simulink model "Wishbone_loads"  (R2024b)
settings: Solver=VariableStepAuto  StartTime=0.0  StopTime=10.0  RelTol=1e-3
libraries: simulink x6
(part 1 of 2)
settings Model: Creator=andre  LastModifiedBy=andre

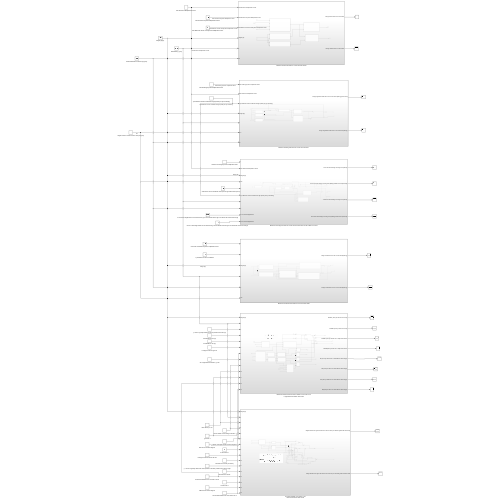
[thumbnail: Simulink's stored preview of the top-level diagram]
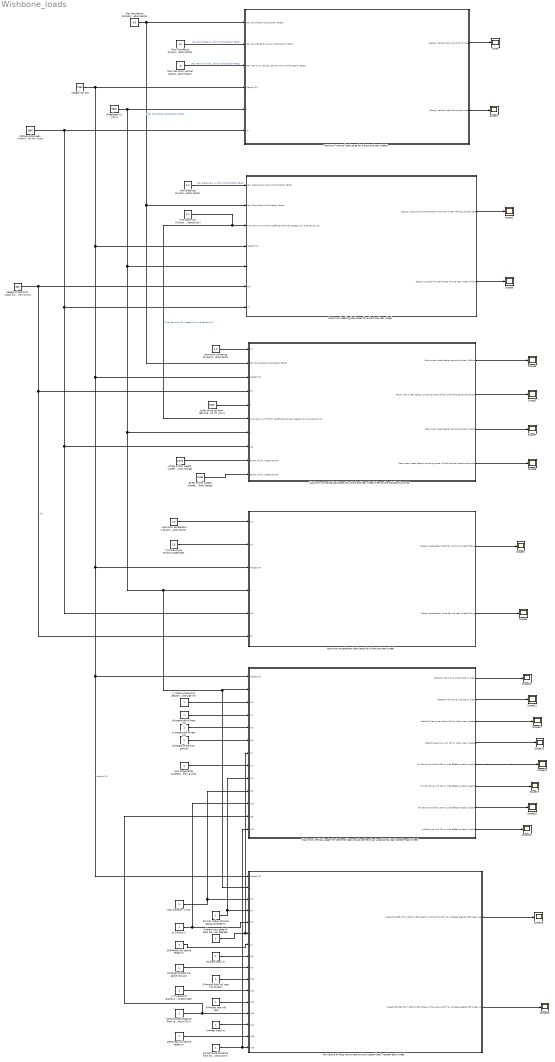
== system Wishbone_loads ==
  37.5% of this weight tranfer can be assumed to go to rear wheels nned to figure out where this comes from though : Constant  Value=0.375
  62.5% of this weight tranfer can be assumed to go to front wheels nned to figure out where this comes from though : Constant  Value=0.625
  Alpha= max angle of bank from floor degrees : Constant
  Ax= longitudinal acceleration  g units : Constant
  Distance Between Front Axle (lm) [mm] : Constant  Value=1950
  For Centre of Mass not at centre of car Lateral load Transfer-each wheel : Subsystem
  H=height of total CG above roll axis : Constant
  Height of centre of mass from the road (Hm) [mm] : Constant  Value=325
  KF=total front roll rate ( lb.-ft/rad?) : Constant
  KR=total rear roll rate : Constant
  Max Breaking Dynamic Multiplication Factor : Constant  Value=1.3
  Max Downforce Dynamic Multiplication Factor : Constant  Value=1.3
  Max Downforce Multiplication Factor : Constant  Value=3.3
  Max Maximum Verical Load Dynamic Multiplication Factor : Constant  Value=3
  Max Velocity- V m/s : Constant
  "Maximum Vertical Loads-For Centre of Mass not at centre of car Longitudinal load transfer-each wheel " : Subsystem
  Maximum acceleraton load cases for a front and rear wheel : Subsystem
  Maximum breaking load cases for a front and rear wheel : Subsystem
  Maximum cornering load cases for a front and rear wheel when on the outside of a corner : Subsystem
  Maximum vertical load cases for a front and rear wheels : Subsystem
  R=max radius of circle being cornered m : Constant
  Scope{,1..19} (20 alike) : Scope
  Tyre Maximum Friction Coefficient : Constant  Value=1.5
  Tyre Maximum Friction Coefficient at high speeds (low tyre sensitivity) : Constant  Value=1.2
  Weight (W) [N] : Constant  Value=7350
  Wheelbase (L) [mm] : Constant  Value=3215
  ZRF=front roll centre height m : Constant
  ZRR=rear roll centre height m : Constant
  a=horizontal distance from front axle to CG m : Constant
  b=horizontal distance from rear axle to CG m : Constant
  g- 9.81ms-2 : Constant
  "h=height of CG from ground " : Constant
  maximum acceleration Dynamic multiplication factor : Constant  Value=1.3
  maximum cornering Dynamic multiplication factor : Constant  Value=1.3
  tf treadwidth of front (m) : Constant
  tf=front track m : Constant
  tr treadwidth of rear (m) : Constant
  tr=rear track m : Constant
  width of the car from left wheel centre point to right wheel centre point (T) [mm] : Constant  Value=1500
  y’’ centre of gravitys offset from centre position to the side (m) : Constant
  "y’’= centre of gravitys offset from centre position to the side, positive when going to right" : Constant
  wires:
  Max Downforce Dynamic Multiplication Factor/1 -> Maximum vertical load cases for a front and rear wheels/2(Max Downforce Dynamic Multiplication Factor)  "Max Downforce Dynamic Multiplication Factor"
  Max Maximum Verical Load Dynamic Multiplication Factor/1 -> Maximum vertical load cases for a front and rear wheels/3(Max Maximum Verical Load Dynamic Multiplication Factor)  "Max Maximum Verical Load Dynamic Multiplication Factor"
  Weight (W) [N]/1 -> Maximum vertical load cases for a front and rear wheels/4(Weight (W)), Maximum breaking load cases for a front and rear wheel/4(Weight (W)), For Centre of Mass not at centre of car Lateral load Transfer-each wheel/1(Weight (W)), "Maximum Vertical Loads-For Centre of Mass not at centre of car Longitudinal load transfer-each wheel "/1(Weight (W)), Maximum acceleraton load cases for a front and rear wheel/3(Weight (W)), Maximum cornering load cases for a front and rear wheel when on the outside of a corner/3(Weight (W))  "Weight (W)"
  Wheelbase (L) [mm]/1 -> For Centre of Mass not at centre of car Lateral load Transfer-each wheel/2(L), "Maximum Vertical Loads-For Centre of Mass not at centre of car Longitudinal load transfer-each wheel "/2(L), Maximum acceleraton load cases for a front and rear wheel/4(L), Maximum cornering load cases for a front and rear wheel when on the outside of a corner/7(L), Maximum breaking load cases for a front and rear wheel/5(L), Maximum vertical load cases for a front and rear wheels/5(L)  "L"
  Distance Between Front Axle (lm) [mm]/1 -> Maximum acceleraton load cases for a front and rear wheel/5(In5), Maximum cornering load cases for a front and rear wheel when on the outside of a corner/8(In8), Maximum breaking load cases for a front and rear wheel/7(lm), Maximum vertical load cases for a front and rear wheels/6(lm)
  Maximum vertical load cases for a front and rear wheels/1(Design Vertical load of one front wheel) -> Scope/1
  Maximum vertical load cases for a front and rear wheels/2(Design Vertical load of one rear wheel) -> Scope4/1
  Max Downforce Multiplication Factor/1 -> Maximum cornering load cases for a front and rear wheel when on the outside of a corner/2(Max Downforce Multiplication Factor), Maximum breaking load cases for a front and rear wheel/2(Max Downforce Multiplication Factor), Maximum vertical load cases for a front and rear wheels/1(Max Downforce Multiplication Factor)  "Max Downforce Multiplication Factor"
  Max Breaking Dynamic Multiplication Factor/1 -> Maximum breaking load cases for a front and rear wheel/1(Max breaking dynamic multiplication factor)  "Max breaking dynamic multiplication factor"
  Tyre Maximum Friction Coefficient at high speeds (low tyre sensitivity)/1 -> Maximum cornering load cases for a front and rear wheel when on the outside of a corner/6(Tyre Maximum Friction Coefficient at high speeds (low tyre sensitivity)), Maximum breaking load cases for a front and rear wheel/3(Tyre Maximum Friction Coefficient at high speeds (low tyre sensitivity))  "Tyre Maximum Friction Coefficient at high speeds (low tyre sensitivity)"
  Height of centre of mass from the road (Hm) [mm]/1 -> Maximum acceleraton load cases for a front and rear wheel/6(Hm), Maximum cornering load cases for a front and rear wheel when on the outside of a corner/4(Hm), Maximum breaking load cases for a front and rear wheel/6(Hm)  "Hm"
  Maximum breaking load cases for a front and rear wheel/1(Design longitudinal brake force for one front wheel (Wflong) [critical case]) -> Scope1/1
  Maximum breaking load cases for a front and rear wheel/2(Design longitudinal brake force for one rear wheel (Wrlong)) -> Scope5/1
  maximum cornering Dynamic multiplication factor/1 -> Maximum cornering load cases for a front and rear wheel when on the outside of a corner/1(In1)
  width of the car from left wheel centre point to right wheel centre point (T) [mm]/1 -> Maximum cornering load cases for a front and rear wheel when on the outside of a corner/5(T)
  Maximum cornering load cases for a front and rear wheel when on the outside of a corner/1(Front outer wheel design cornering force (Wfolat)) -> Scope6/1
  Maximum cornering load cases for a front and rear wheel when on the outside of a corner/4(Rear outer wheel design cornering force (Wrilat) [smaller force expericned]) -> Scope8/1
  Maximum cornering load cases for a front and rear wheel when on the outside of a corner/3(Rear outer wheel design cornering force (Wrolat)) -> Scope7/1
  Maximum cornering load cases for a front and rear wheel when on the outside of a corner/2(Front inner wheel design cornering force (Wfilat) [smaller forces experienced]) -> Scope2/1
  maximum acceleration Dynamic multiplication factor/1 -> Maximum acceleraton load cases for a front and rear wheel/1(In1)
  Tyre Maximum Friction Coefficient/1 -> Maximum acceleraton load cases for a front and rear wheel/2(In2)
  Maximum acceleraton load cases for a front and rear wheel/1(Design acceleration force for one front wheel(Wflong)) -> Scope3/1
  Maximum acceleraton load cases for a front and rear wheel/2(Design acceleration force for one rear wheel(Wrlong)) -> Scope9/1
  37.5% of this weight tranfer can be assumed to go to rear wheels nned to figure out where this comes from though/1 -> Maximum cornering load cases for a front and rear wheel when on the outside of a corner/9("37.5% of this weight tranfer ")
  62.5% of this weight tranfer can be assumed to go to front wheels nned to figure out where this comes from though/1 -> Maximum cornering load cases for a front and rear wheel when on the outside of a corner/10(62.5% of this weight tranfer)
  y’’ centre of gravitys offset from centre position to the side (m)/1 -> "Maximum Vertical Loads-For Centre of Mass not at centre of car Longitudinal load transfer-each wheel "/3(In3)
  tf treadwidth of front (m)/1 -> "Maximum Vertical Loads-For Centre of Mass not at centre of car Longitudinal load transfer-each wheel "/4(In4)
  tr treadwidth of rear (m)/1 -> "Maximum Vertical Loads-For Centre of Mass not at centre of car Longitudinal load transfer-each wheel "/5(In5)
  "h=height of CG from ground "/1 -> "Maximum Vertical Loads-For Centre of Mass not at centre of car Longitudinal load transfer-each wheel "/6(In6)
  Ax= longitudinal acceleration  g units/1 -> "Maximum Vertical Loads-For Centre of Mass not at centre of car Longitudinal load transfer-each wheel "/8(In7)
  "Maximum Vertical Loads-For Centre of Mass not at centre of car Longitudinal load transfer-each wheel "/1(DeltaW1 (front tyre without CG on side)) -> Scope10/1
  "Maximum Vertical Loads-For Centre of Mass not at centre of car Longitudinal load transfer-each wheel "/2(DeltaW2 (front tyre with CG on side)) -> Scope11/1
  "Maximum Vertical Loads-For Centre of Mass not at centre of car Longitudinal load transfer-each wheel "/3(DeltaW3 (rear tyre without CG on side) load increase) -> Scope12/1
  "Maximum Vertical Loads-For Centre of Mass not at centre of car Longitudinal load transfer-each wheel "/4(DeltaW4(rear tyre with CG on side) load increase) -> Scope13/1
  Max Velocity- V m/s/1 -> "Maximum Vertical Loads-For Centre of Mass not at centre of car Longitudinal load transfer-each wheel "/10(In9), For Centre of Mass not at centre of car Lateral load Transfer-each wheel/3(In3)
  R=max radius of circle being cornered m/1 -> "Maximum Vertical Loads-For Centre of Mass not at centre of car Longitudinal load transfer-each wheel "/9(In2), For Centre of Mass not at centre of car Lateral load Transfer-each wheel/4(In4)
  Alpha= max angle of bank from floor degrees/1 -> "Maximum Vertical Loads-For Centre of Mass not at centre of car Longitudinal load transfer-each wheel "/7(In1), For Centre of Mass not at centre of car Lateral load Transfer-each wheel/6(u)
  ZRF=front roll centre height m/1 -> For Centre of Mass not at centre of car Lateral load Transfer-each wheel/7(In7)
  tf=front track m/1 -> For Centre of Mass not at centre of car Lateral load Transfer-each wheel/8(In8)
  H=height of total CG above roll axis/1 -> For Centre of Mass not at centre of car Lateral load Transfer-each wheel/9(In9)
  KF=total front roll rate ( lb.-ft/rad?)/1 -> For Centre of Mass not at centre of car Lateral load Transfer-each wheel/10(In10)
  "y’’= centre of gravitys offset from centre position to the side, positive when going to right"/1 -> For Centre of Mass not at centre of car Lateral load Transfer-each wheel/11(In11)
  KR=total rear roll rate/1 -> For Centre of Mass not at centre of car Lateral load Transfer-each wheel/12(In12)
  b=horizontal distance from rear axle to CG m/1 -> "Maximum Vertical Loads-For Centre of Mass not at centre of car Longitudinal load transfer-each wheel "/12(In8), For Centre of Mass not at centre of car Lateral load Transfer-each wheel/13(In13)
  tr=rear track m/1 -> For Centre of Mass not at centre of car Lateral load Transfer-each wheel/14(In14)
  ZRR=rear roll centre height m/1 -> For Centre of Mass not at centre of car Lateral load Transfer-each wheel/15(In15)
  For Centre of Mass not at centre of car Lateral load Transfer-each wheel/1(Weight transfer from right to left wheel on the front axle(+ve indicates greater left wheel load)) -> Scope18/1
  For Centre of Mass not at centre of car Lateral load Transfer-each wheel/2(Weight transfer from right to left wheel on the rear axle(+ve indicates greater left wheel load) -> Scope19/1
  g- 9.81ms-2/1 -> "Maximum Vertical Loads-For Centre of Mass not at centre of car Longitudinal load transfer-each wheel "/11(In11), For Centre of Mass not at centre of car Lateral load Transfer-each wheel/5(In5)
  a=horizontal distance from front axle to CG m/1 -> "Maximum Vertical Loads-For Centre of Mass not at centre of car Longitudinal load transfer-each wheel "/13(In12), For Centre of Mass not at centre of car Lateral load Transfer-each wheel/16(In16)
  "Maximum Vertical Loads-For Centre of Mass not at centre of car Longitudinal load transfer-each wheel "/5(W1 (front tyre without CG on side Effective static weight)) -> Scope14/1
  "Maximum Vertical Loads-For Centre of Mass not at centre of car Longitudinal load transfer-each wheel "/6(W2 (front tyre with CG on side effective static weight)) -> Scope17/1
  "Maximum Vertical Loads-For Centre of Mass not at centre of car Longitudinal load transfer-each wheel "/7(W3 (rear tyre without CG on side effective static weight)) -> Scope16/1
  "Maximum Vertical Loads-For Centre of Mass not at centre of car Longitudinal load transfer-each wheel "/8(W4(rear tyre with CG on side effective static weight)) -> Scope15/1

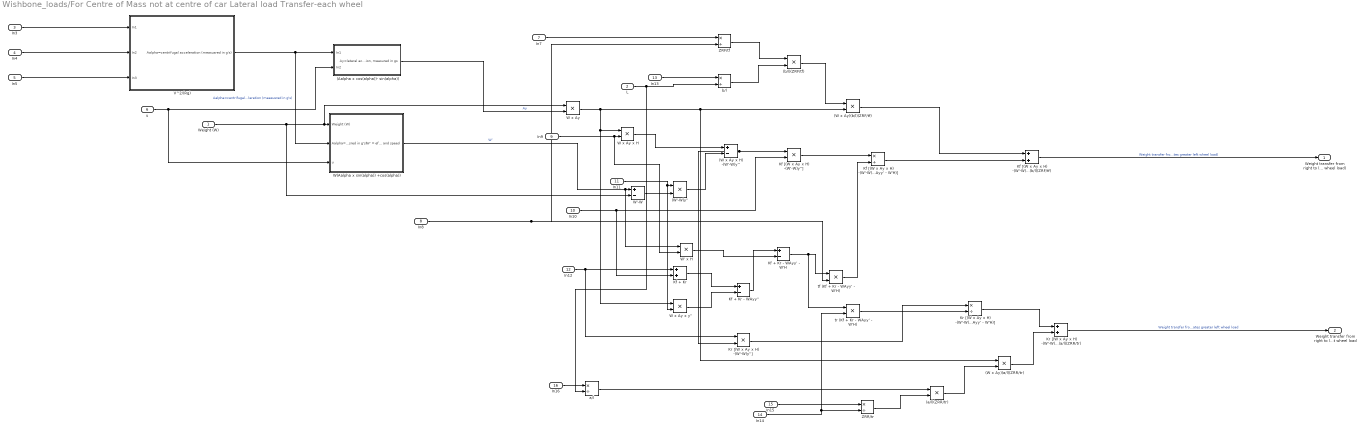
== system Wishbone_loads/For Centre of Mass not at centre of car Lateral load Transfer-each wheel ==
  Weight (W) : Inport
  L : Inport  Port=2
  In3 : Inport  Port=3
  In4 : Inport  Port=4
  In5 : Inport  Port=5
  u : Inport  Port=6
  In7 : Inport  Port=7
  In8 : Inport  Port=8
  In9 : Inport  Port=9
  In10 : Inport  Port=10
  In11 : Inport  Port=11
  In12 : Inport  Port=12
  In13 : Inport  Port=13
  In14 : Inport  Port=14
  In15 : Inport  Port=15
  In16 : Inport  Port=16
  (Aalpha x cos(alpha))- sin(alpha)) : Subsystem
  (W x Ay x H) -(W'-W)y'' : Sum  Inputs=+-
  (W x Ay)(a/l)(ZRR/tr) : Product
  (W x Ay)(b/l)(ZRF/tf) : Product
  (W'-W)y'' : Product
  (a/l)(ZRR/tr) : Product
  (b/l)(ZRF/tf) : Product
  Kf + Kr : Sum
  Kf + Kr - WAyy' - W'H : Sum  Inputs=+-
  Kf + Kr - WAyy'' : Sum  Inputs=+-
  Kf [(W x Ay x H) -(W'-W)y''] : Product
  Kf [(W x Ay x H) -(W'-W)y''] / [tf (Kf + Kr - WAyy' - W'H)] : Product  Inputs=*/
  Kf [(W x Ay x H) -(W'-W)y''] / [tf (Kf + Kr - WAyy' - W'H)] + (W x Ay)(b/l)(ZRF/tf) : Sum
  Kr [(W x Ay x H) -(W'-W)y''] : Product
  Kr [(W x Ay x H) -(W'-W)y''] / [tr (Kf + Kr - WAyy' - W'H)] : Product  Inputs=*/
  Kr [(W x Ay x H) -(W'-W)y''] / [tr (Kf + Kr - WAyy' - W'H)]/ (W x Ay)(a/l)(ZRR/tr) : Sum
  V^2/(Rg) : Subsystem
  W x Ay : Product
  W x Ay x H : Product
  W x Ay x y'' : Product
  W' x H : Product
  W'-W : Sum  Inputs=+-
  W(Aalpha x sin(alpha)) +cos(alpha)) : Subsystem
  ZRF/tf : Product  Inputs=*/
  ZRR/tr : Product  Inputs=*/
  a/l : Product  Inputs=*/
  b/l : Product  Inputs=*/
  tf (Kf + Kr - WAyy' - W'H) : Product
  tr (Kf + Kr - WAyy' - W'H) : Product
  Weight transfer from right to left wheel on the front axle(+ve indicates greater left wheel load) : Outport
  Weight transfer from right to left wheel on the rear axle(+ve indicates greater left wheel load : Outport  Port=2
  wires:
  Kr [(W x Ay x H) -(W'-W)y'']/1 -> Kr [(W x Ay x H) -(W'-W)y''] / [tr (Kf + Kr - WAyy' - W'H)]/1
  ZRR/tr/1 -> (a/l)(ZRR/tr)/2
  Weight (W)/1 -> W'-W/2, W x Ay/1, W(Aalpha x sin(alpha)) +cos(alpha))/1(Weight (W))
  In5/1 -> V^2/(Rg)/3(In3)
  Kf [(W x Ay x H) -(W'-W)y'']/1 -> Kf [(W x Ay x H) -(W'-W)y''] / [tf (Kf + Kr - WAyy' - W'H)]/1
  V^2/(Rg)/1(Aalpha=centrifugal acceleration (measusred in g's)) -> W(Aalpha x sin(alpha)) +cos(alpha))/2(Aalpha=centrifugal acceleration (measusred in g's)), (Aalpha x cos(alpha))- sin(alpha))/1(In1)  "Aalpha=centrifugal acceleration (measusred in g's)"
  W x Ay/1 -> W x Ay x y''/1, W x Ay x H/1, (W x Ay)(a/l)(ZRR/tr)/1, (W x Ay)(b/l)(ZRF/tf)/2
  W x Ay x H/1 -> (W x Ay x H) -(W'-W)y''/1
  Kf + Kr - WAyy' - W'H/1 -> tf (Kf + Kr - WAyy' - W'H)/1, tr (Kf + Kr - WAyy' - W'H)/1
  (Aalpha x cos(alpha))- sin(alpha))/1("Ay=lateral acceleration, measured in gs") -> W x Ay/2  "Ay"
  (b/l)(ZRF/tf)/1 -> (W x Ay)(b/l)(ZRF/tf)/1
  In10/1 -> Kf + Kr/2, Kf [(W x Ay x H) -(W'-W)y'']/2
  (W x Ay)(a/l)(ZRR/tr)/1 -> Kr [(W x Ay x H) -(W'-W)y''] / [tr (Kf + Kr - WAyy' - W'H)]/ (W x Ay)(a/l)(ZRR/tr)/2
  In12/1 -> Kr [(W x Ay x H) -(W'-W)y'']/1, Kf + Kr/1
  W' x H/1 -> Kf + Kr - WAyy' - W'H/2
  Kf + Kr - WAyy''/1 -> Kf + Kr - WAyy' - W'H/1
  W(Aalpha x sin(alpha)) +cos(alpha))/1(W’ = effective weight due to bank angle and speed) -> W' x H/1, W'-W/1  "W’"
  L/1 -> a/l/2, b/l/2
  Kr [(W x Ay x H) -(W'-W)y''] / [tr (Kf + Kr - WAyy' - W'H)]/1 -> Kr [(W x Ay x H) -(W'-W)y''] / [tr (Kf + Kr - WAyy' - W'H)]/ (W x Ay)(a/l)(ZRR/tr)/1
  (a/l)(ZRR/tr)/1 -> (W x Ay)(a/l)(ZRR/tr)/2
  In8/1 -> tf (Kf + Kr - WAyy' - W'H)/2, ZRF/tf/2
  u/1 -> W(Aalpha x sin(alpha)) +cos(alpha))/3(u), (Aalpha x cos(alpha))- sin(alpha))/2(In2)
  W x Ay x y''/1 -> Kf + Kr - WAyy''/2
  In14/1 -> tr (Kf + Kr - WAyy' - W'H)/2, ZRR/tr/2
  W'-W/1 -> (W'-W)y''/2
  (W x Ay)(b/l)(ZRF/tf)/1 -> Kf [(W x Ay x H) -(W'-W)y''] / [tf (Kf + Kr - WAyy' - W'H)] + (W x Ay)(b/l)(ZRF/tf)/1
  tr (Kf + Kr - WAyy' - W'H)/1 -> Kr [(W x Ay x H) -(W'-W)y''] / [tr (Kf + Kr - WAyy' - W'H)]/2
  In11/1 -> W x Ay x y''/2, (W'-W)y''/1
  In15/1 -> ZRR/tr/1
  In9/1 -> W' x H/2, W x Ay x H/2
  (W'-W)y''/1 -> (W x Ay x H) -(W'-W)y''/2
  Kf [(W x Ay x H) -(W'-W)y''] / [tf (Kf + Kr - WAyy' - W'H)]/1 -> Kf [(W x Ay x H) -(W'-W)y''] / [tf (Kf + Kr - WAyy' - W'H)] + (W x Ay)(b/l)(ZRF/tf)/2
  tf (Kf + Kr - WAyy' - W'H)/1 -> Kf [(W x Ay x H) -(W'-W)y''] / [tf (Kf + Kr - WAyy' - W'H)]/2
  b/l/1 -> (b/l)(ZRF/tf)/2
  In3/1 -> V^2/(Rg)/1(In1)
  (W x Ay x H) -(W'-W)y''/1 -> Kr [(W x Ay x H) -(W'-W)y'']/2, Kf [(W x Ay x H) -(W'-W)y'']/1
  In7/1 -> ZRF/tf/1
  Kf + Kr/1 -> Kf + Kr - WAyy''/1
  In4/1 -> V^2/(Rg)/2(In2)
  ZRF/tf/1 -> (b/l)(ZRF/tf)/1
  Kr [(W x Ay x H) -(W'-W)y''] / [tr (Kf + Kr - WAyy' - W'H)]/ (W x Ay)(a/l)(ZRR/tr)/1 -> Weight transfer from right to left wheel on the rear axle(+ve indicates greater left wheel load/1  "Weight transfer from right to left wheel on the rear axle(+ve indicates greater left wheel load"
  In13/1 -> b/l/1
  Kf [(W x Ay x H) -(W'-W)y''] / [tf (Kf + Kr - WAyy' - W'H)] + (W x Ay)(b/l)(ZRF/tf)/1 -> Weight transfer from right to left wheel on the front axle(+ve indicates greater left wheel load)/1  "Weight transfer from right to left wheel on the front axle(+ve indicates greater left wheel load)"
  In16/1 -> a/l/1
  a/l/1 -> (a/l)(ZRR/tr)/1

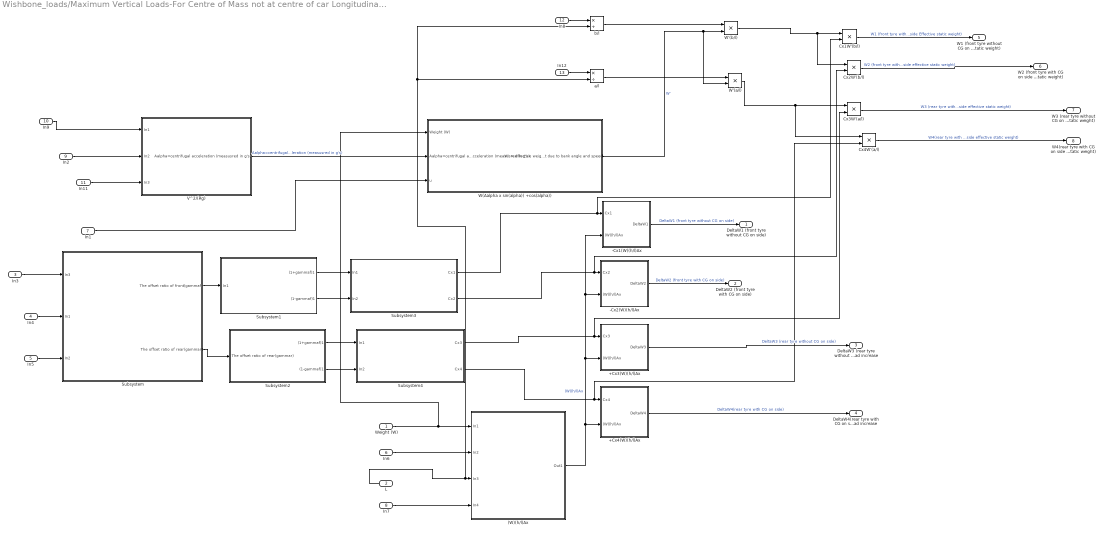
== system Wishbone_loads/Maximum Vertical Loads-For Centre of Mass not at centre of car Longitudinal load transfer-each wheel  ==
  Weight (W) : Inport
  L : Inport  Port=2
  In3 : Inport  Port=3
  In4 : Inport  Port=4
  In5 : Inport  Port=5
  In6 : Inport  Port=6
  In1 : Inport  Port=7
  In7 : Inport  Port=8
  In2 : Inport  Port=9
  In9 : Inport  Port=10
  In11 : Inport  Port=11
  In8 : Inport  Port=12
  In12 : Inport  Port=13
  (W)(h/l)Ax : Subsystem
  +Cx3(W)(h/l)Ax : Subsystem
  "+Cx4(W)(h/l)Ax " : Subsystem
  -Cx1(W)(h/l)Ax : Subsystem
  "-Cx2(W)(h/l)Ax " : Subsystem
  Cx1W'(b/l) : Product
  Cx2W'(b/l) : Product
  Cx3W'(a/l) : Product
  Cx4W'(a/l) : Product
  Subsystem : Subsystem
  Subsystem1 : Subsystem
  Subsystem2 : Subsystem
  Subsystem3 : Subsystem
  Subsystem4 : Subsystem
  V^2/(Rg) : Subsystem
  W'(a/l) : Product
  W'(b/l) : Product
  W(Aalpha x sin(alpha)) +cos(alpha)) : Subsystem
  a/l : Product  Inputs=*/
  b/l : Product  Inputs=*/
  DeltaW1 (front tyre without CG on side) : Outport
  DeltaW2 (front tyre with CG on side) : Outport  Port=2
  DeltaW3 (rear tyre without CG on side) load increase : Outport  Port=3
  DeltaW4(rear tyre with CG on side) load increase : Outport  Port=4
  W1 (front tyre without CG on side Effective static weight) : Outport  Port=5
  W2 (front tyre with CG on side effective static weight) : Outport  Port=6
  W3 (rear tyre without CG on side effective static weight) : Outport  Port=7
  W4(rear tyre with CG on side effective static weight) : Outport  Port=8
  wires:
  Weight (W)/1 -> W(Aalpha x sin(alpha)) +cos(alpha))/1(Weight (W)), (W)(h/l)Ax/1(In1)
  Subsystem4/2(Cx4) -> Cx4W'(a/l)/2, "+Cx4(W)(h/l)Ax "/1(Cx4)
  Subsystem/2(The offset ratio of rear(gammar)) -> Subsystem2/1(The offset ratio of rear(gammar))
  (W)(h/l)Ax/1(Out1) -> -Cx1(W)(h/l)Ax/2((W)(h/l)Ax), "-Cx2(W)(h/l)Ax "/2((W)(h/l)Ax), +Cx3(W)(h/l)Ax/2((W)(h/l)Ax), "+Cx4(W)(h/l)Ax "/2((W)(h/l)Ax)  "(W)(h/l)Ax"
  Subsystem1/1((1+gammaf)1) -> Subsystem3/1(In1)
  Subsystem2/2((1-gammaf)1) -> Subsystem4/2(In2)
  Subsystem3/1(Cx1) -> Cx1W'(b/l)/2, -Cx1(W)(h/l)Ax/1(Cx1)
  Subsystem/1(The offset ratio of front(gammaf)) -> Subsystem1/1(In1)
  "+Cx4(W)(h/l)Ax "/1(DeltaW4) -> DeltaW4(rear tyre with CG on side) load increase/1  "DeltaW4(rear tyre with CG on side)"
  +Cx3(W)(h/l)Ax/1(DeltaW3) -> DeltaW3 (rear tyre without CG on side) load increase/1  "DeltaW3 (rear tyre without CG on side)"
  Subsystem1/2((1-gammaf)1) -> Subsystem3/2(In2)
  Subsystem3/2(Cx2) -> Cx2W'(b/l)/2, "-Cx2(W)(h/l)Ax "/1(Cx2)
  Subsystem4/1(Cx3) -> Cx3W'(a/l)/2, +Cx3(W)(h/l)Ax/1(Cx3)
  In7/1 -> (W)(h/l)Ax/4(In4)
  Subsystem2/1((1+gammaf)1) -> Subsystem4/1(In1)
  -Cx1(W)(h/l)Ax/1(DeltaW1) -> DeltaW1 (front tyre without CG on side)/1  "DeltaW1 (front tyre without CG on side)"
  L/1 -> b/l/2, a/l/2, (W)(h/l)Ax/3(In3)
  In3/1 -> Subsystem/1(In3)
  "-Cx2(W)(h/l)Ax "/1(DeltaW2) -> DeltaW2 (front tyre with CG on side)/1  "DeltaW2 (front tyre with CG on side)"
  In6/1 -> (W)(h/l)Ax/2(In2)
  In4/1 -> Subsystem/2(In1)
  In5/1 -> Subsystem/3(In2)
  W(Aalpha x sin(alpha)) +cos(alpha))/1(W’ = effective weight due to bank angle and speed) -> W'(a/l)/2, W'(b/l)/2  "W’"
  V^2/(Rg)/1(Aalpha=centrifugal acceleration (measusred in g's)) -> W(Aalpha x sin(alpha)) +cos(alpha))/2(Aalpha=centrifugal acceleration (measusred in g's))  "Aalpha=centrifugal acceleration (measusred in g's)"
  In1/1 -> W(Aalpha x sin(alpha)) +cos(alpha))/3(u)
  In9/1 -> V^2/(Rg)/1(In1)
  In2/1 -> V^2/(Rg)/2(In2)
  In11/1 -> V^2/(Rg)/3(In3)
  In12/1 -> a/l/1
  In8/1 -> b/l/1
  b/l/1 -> W'(b/l)/1
  a/l/1 -> W'(a/l)/1
  W'(b/l)/1 -> Cx1W'(b/l)/1, Cx2W'(b/l)/1
  W'(a/l)/1 -> Cx3W'(a/l)/1, Cx4W'(a/l)/1
  Cx2W'(b/l)/1 -> W2 (front tyre with CG on side effective static weight)/1  "W2 (front tyre with CG on side effective static weight)"
  Cx3W'(a/l)/1 -> W3 (rear tyre without CG on side effective static weight)/1  "W3 (rear tyre without CG on side effective static weight)"
  Cx4W'(a/l)/1 -> W4(rear tyre with CG on side effective static weight)/1  "W4(rear tyre with CG on side effective static weight)"
  Cx1W'(b/l)/1 -> W1 (front tyre without CG on side Effective static weight)/1  "W1 (front tyre without CG on side Effective static weight)"

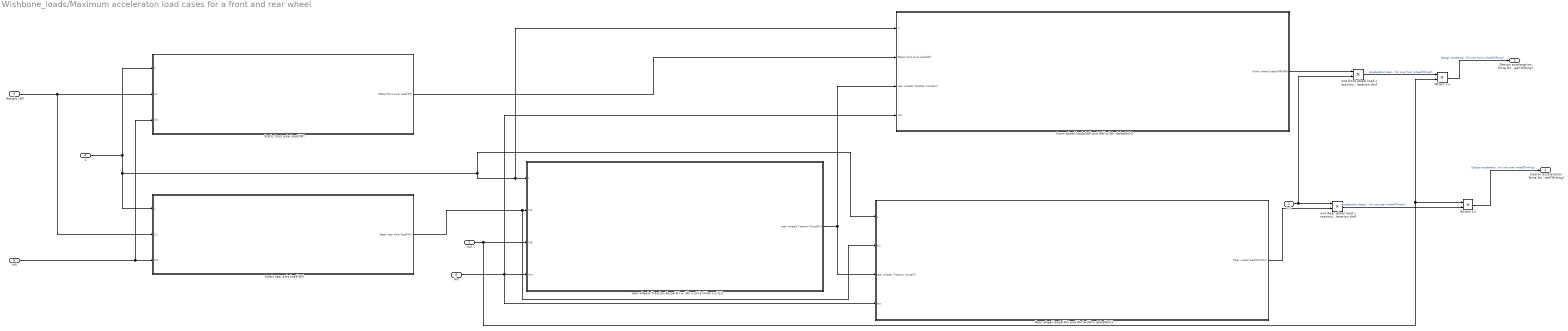
== system Wishbone_loads/Maximum acceleraton load cases for a front and rear wheel ==
  In1 : Inport
  In2 : Inport  Port=2
  Weight (W) : Inport  Port=3
  L : Inport  Port=4
  In5 : Inport  Port=5
  Hm : Inport  Port=6
  Front wheel loads(Wfl and Wfr)=(Wr- deltaWx)/2 : Subsystem
  Rear wheel loads(Wrl and Wrr)=(Wr+ deltaWx)/2 : Subsystem
  Static front axle load(Wf) : Subsystem
  Static rear axle load(Wr) : Subsystem
  Wfvert x u : Product
  Wrvert x u : Product
  one Rear wheel load x maximum acceleration dmf : Product
  one front wheel load x maximum acceleration dmf : Product
  rear wheels Traction Force(Fr) = (Wr x u)/[1-((Hm x u)/L)] : Subsystem
  Design acceleration force for one front wheel(Wflong) : Outport
  Design acceleration force for one rear wheel(Wrlong) : Outport  Port=2
  wires:
  one front wheel load x maximum acceleration dmf/1 -> Wfvert x u/1  "Acceleration design load for one front wheel(Wfvert)"
  Front wheel loads(Wfl and Wfr)=(Wr- deltaWx)/2/1(Front wheel loads(Wfl/Wfr)) -> one front wheel load x maximum acceleration dmf/1
  In2/1 -> Wfvert x u/2, Wrvert x u/1, rear wheels Traction Force(Fr) = (Wr x u)/[1-((Hm x u)/L)]/3(In3)
  L/1 -> Rear wheel loads(Wrl and Wrr)=(Wr+ deltaWx)/2/1(L), rear wheels Traction Force(Fr) = (Wr x u)/[1-((Hm x u)/L)]/1(L), Front wheel loads(Wfl and Wfr)=(Wr- deltaWx)/2/1(L), Static rear axle load(Wr)/1(L), Static front axle load(Wf)/1(L)
  Rear wheel loads(Wrl and Wrr)=(Wr+ deltaWx)/2/1(Rear wheel load(Wrl/Wrr)) -> one Rear wheel load x maximum acceleration dmf/2
  Hm/1 -> rear wheels Traction Force(Fr) = (Wr x u)/[1-((Hm x u)/L)]/4(Hm), Front wheel loads(Wfl and Wfr)=(Wr- deltaWx)/2/4(Hm), Rear wheel loads(Wrl and Wrr)=(Wr+ deltaWx)/2/4(Hm)
  Static rear axle load(Wr)/1(Static rear axle load(Wr)) -> Rear wheel loads(Wrl and Wrr)=(Wr+ deltaWx)/2/2(In2), rear wheels Traction Force(Fr) = (Wr x u)/[1-((Hm x u)/L)]/2(In2)
  In5/1 -> Static rear axle load(Wr)/3(In3), Static front axle load(Wf)/3(In3)
  rear wheels Traction Force(Fr) = (Wr x u)/[1-((Hm x u)/L)]/1(rear wheels Traction Force(Fr)) -> Front wheel loads(Wfl and Wfr)=(Wr- deltaWx)/2/3(rear wheels Traction Force(Fr)), Rear wheel loads(Wrl and Wrr)=(Wr+ deltaWx)/2/3(rear wheels Traction Force(F))
  Static front axle load(Wf)/1(Static front axle load(Wf)) -> Front wheel loads(Wfl and Wfr)=(Wr- deltaWx)/2/2(Static front axle load(Wf))
  one Rear wheel load x maximum acceleration dmf/1 -> Wrvert x u/2  "Acceleration design load for one rear wheel(Wrvert)"
  Weight (W)/1 -> Static front axle load(Wf)/2(L1), Static rear axle load(Wr)/2(L1)
  In1/1 -> one Rear wheel load x maximum acceleration dmf/1, one front wheel load x maximum acceleration dmf/2
  Wrvert x u/1 -> Design acceleration force for one rear wheel(Wrlong)/1  "Design acceleration force for one rear wheel(Wrlong)"
  Wfvert x u/1 -> Design acceleration force for one front wheel(Wflong)/1  "Design acceleration force for one front wheel(Wflong)"

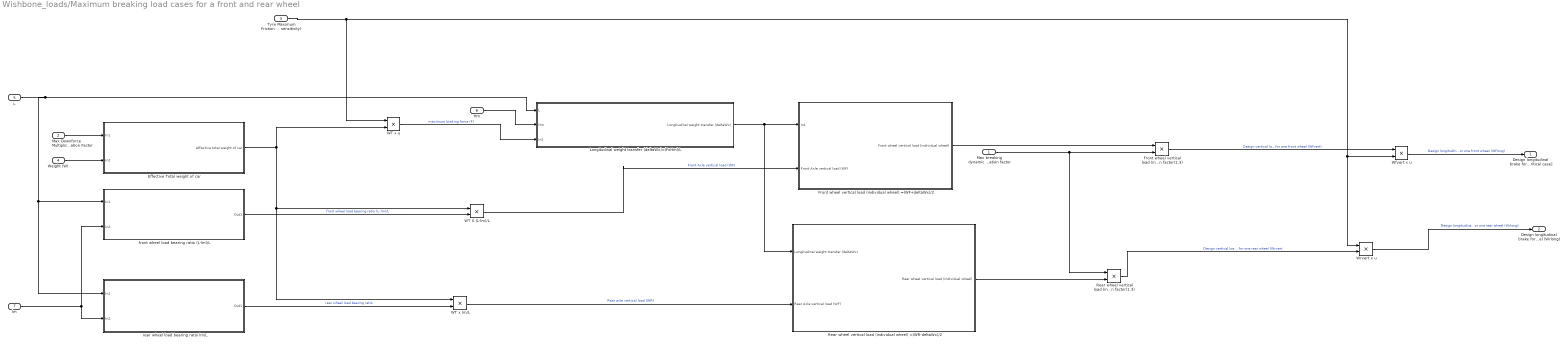
== system Wishbone_loads/Maximum breaking load cases for a front and rear wheel ==
  Max breaking dynamic multiplication factor : Inport
  Max Downforce Multiplication Factor : Inport  Port=2
  Tyre Maximum Friction Coefficient at high speeds (low tyre sensitivity) : Inport  Port=3
  Weight (W) : Inport  Port=4
  L : Inport  Port=5
  Hm : Inport  Port=6
  lm : Inport  Port=7
  " WT x lm/L" : Product
  " Wfvert x u" : Product
  " Wrvert x u" : Product
  Effective Total weight of car : Subsystem
  Front wheel vertical load (individual wheel) =(WF+deltaWx)/2 : Subsystem
  Front wheel vertical load (individual wheel) x max breaking dynamic multtiplication factor(1.3) : Product
  Longitudinal weight transfer (deltaWx)=(FxHm)/L : Subsystem
  Rear wheel vertical load (individual wheel) =(WR-deltaWx)/2 : Subsystem
  Rear wheel vertical load (individual wheel) x max breaking dynamic multtiplication factor(1.3) : Product
  WT X (L-lm)/L : Product
  WT x u : Product
  front wheel load bearing ratio (L-lm)/L : Subsystem
  rear wheel load bearing ratio lm/L : Subsystem
  Design longitudinal brake force for one front wheel (Wflong) [critical case] : Outport
  Design longitudinal brake force for one rear wheel (Wrlong) : Outport  Port=2
  wires:
  Max breaking dynamic multiplication factor/1 -> Front wheel vertical load (individual wheel) x max breaking dynamic multtiplication factor(1.3)/2, Rear wheel vertical load (individual wheel) x max breaking dynamic multtiplication factor(1.3)/1
  Tyre Maximum Friction Coefficient at high speeds (low tyre sensitivity)/1 -> WT x u/1, " Wfvert x u"/2, " Wrvert x u"/1
  front wheel load bearing ratio (L-lm)/L/1(Out1) -> WT X (L-lm)/L/2  "front wheel load bearing ratio (L-lm)/L"
  Effective Total weight of car/1(effective total weight of car) -> WT x u/2, " WT x lm/L"/1, WT X (L-lm)/L/1
  Front wheel vertical load (individual wheel) =(WF+deltaWx)/2/1(Front wheel vertical load (individual wheel)) -> Front wheel vertical load (individual wheel) x max breaking dynamic multtiplication factor(1.3)/1
  Front wheel vertical load (individual wheel) x max breaking dynamic multtiplication factor(1.3)/1 -> " Wfvert x u"/1  "Design vertical load for one front wheel (Wfvert)"
  rear wheel load bearing ratio lm/L/1(Out1) -> " WT x lm/L"/2  "rear wheel load bearing ratio"
  L/1 -> front wheel load bearing ratio (L-lm)/L/1(In1), rear wheel load bearing ratio lm/L/1(In1), Longitudinal weight transfer (deltaWx)=(FxHm)/L/1(L)
  WT x u/1 -> Longitudinal weight transfer (deltaWx)=(FxHm)/L/3(In2)  "maximum braking force (F)"
  WT X (L-lm)/L/1 -> Front wheel vertical load (individual wheel) =(WF+deltaWx)/2/2(Front Axle vertical load (WF))  "Front Axle vertical load (WF)"
  Longitudinal weight transfer (deltaWx)=(FxHm)/L/1(Longitudinal weight transfer (deltaWx)) -> Rear wheel vertical load (individual wheel) =(WR-deltaWx)/2/1(Longitudinal weight transfer (deltaWx)), Front wheel vertical load (individual wheel) =(WF+deltaWx)/2/1(In1)
  lm/1 -> front wheel load bearing ratio (L-lm)/L/2(In2), rear wheel load bearing ratio lm/L/2(In2)
  " WT x lm/L"/1 -> Rear wheel vertical load (individual wheel) =(WR-deltaWx)/2/2(Rear Axle vertical load (WF))  "Rear axle vertical load (WR)"
  " Wrvert x u"/1 -> Design longitudinal brake force for one rear wheel (Wrlong)/1  "Design longitudinal brake force for one rear wheel (Wrlong)"
  " Wfvert x u"/1 -> Design longitudinal brake force for one front wheel (Wflong) [critical case]/1  "Design longitudinal brake force for one front wheel (Wflong)"
  Rear wheel vertical load (individual wheel) x max breaking dynamic multtiplication factor(1.3)/1 -> " Wrvert x u"/2  "Design vertical load for one rear wheel (Wrvert"
  Rear wheel vertical load (individual wheel) =(WR-deltaWx)/2/1(Rear wheel vertical load (individual wheel)) -> Rear wheel vertical load (individual wheel) x max breaking dynamic multtiplication factor(1.3)/2
  Max Downforce Multiplication Factor/1 -> Effective Total weight of car/1(In1)
  Weight (W)/1 -> Effective Total weight of car/2(In2)
  Hm/1 -> Longitudinal weight transfer (deltaWx)=(FxHm)/L/2(Hm)

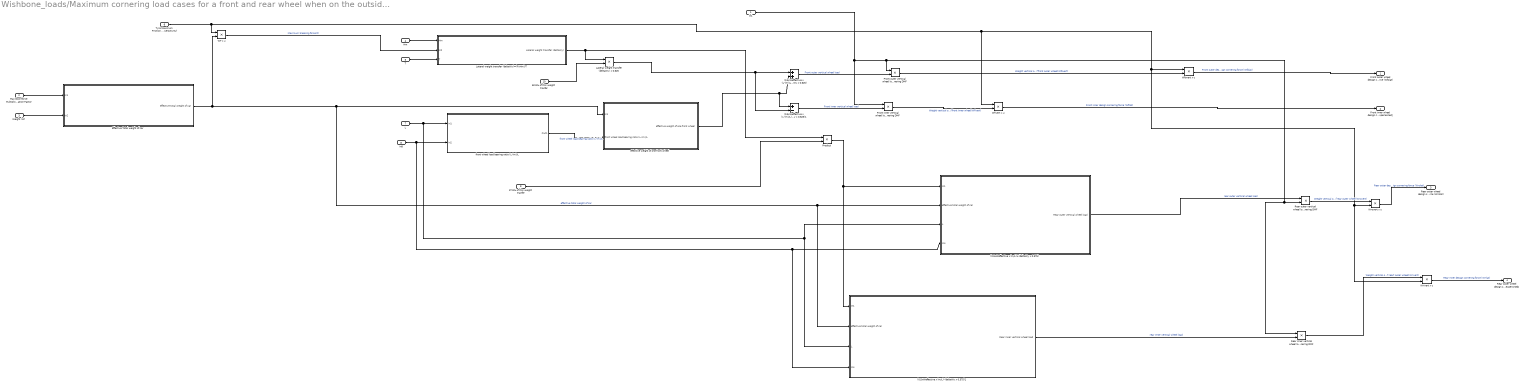
== system Wishbone_loads/Maximum cornering load cases for a front and rear wheel when on the outside of a corner ==
  In1 : Inport
  Max Downforce Multiplication Factor : Inport  Port=2
  Weight (W) : Inport  Port=3
  Hm : Inport  Port=4
  T : Inport  Port=5
  Tyre Maximum Friction Coefficient at high speeds (low tyre sensitivity) : Inport  Port=6
  L : Inport  Port=7
  In8 : Inport  Port=8
  "37.5% of this weight tranfer " : Inport  Port=9
  62.5% of this weight tranfer : Inport  Port=10
  (0.5xWeffective x (L-lm)/L)+(deltaWy x 0.625) : Sum
  (0.5xWeffective x (L-lm)/L)-(deltaWy x 0.625)1 : Sum  Inputs=+-
  (0.5xWeffective x lm/L)+(deltaWy x 0.375) : Subsystem
  (0.5xWeffective x lm/L)-(deltaWy x 0.375)1 : Subsystem
  Effective Total weight of car : Subsystem
  Front inner vertical wheel load x maximum cornering DMF : Product
  Front outer vertical wheel load x maximum cornering DMF : Product
  Lateral weight transfer (deltaWy) x 0.625 : Product
  Lateral weight transfer (deltaWy)=(FxHm)/T : Subsystem
  Product : Product
  Rear inner vertical wheel load x maximum cornering DMF : Product
  Rear outer vertical wheel load x maximum cornering DMF : Product
  WT x u : Product
  Wfivert x u : Product
  Wfovert x u : Product
  Wrivert x u : Product
  Wrovert x u : Product
  effective weight of one front wheel : Subsystem
  front wheel load bearing ratio (L-lm)/L : Subsystem
  Front outer wheel design cornering force (Wfolat) : Outport
  Front inner wheel design cornering force (Wfilat) [smaller forces experienced] : Outport  Port=2
  Rear outer wheel design cornering force (Wrolat) : Outport  Port=3
  Rear outer wheel design cornering force (Wrilat) [smaller force expericned] : Outport  Port=4
  wires:
  In8/1 -> (0.5xWeffective x lm/L)-(deltaWy x 0.375)1/4(In4), (0.5xWeffective x lm/L)+(deltaWy x 0.375)/4(In4), front wheel load bearing ratio (L-lm)/L/2(In2)
  Tyre Maximum Friction Coefficient at high speeds (low tyre sensitivity)/1 -> Wfivert x u/1, Wrivert x u/2, Wrovert x u/2, Wfovert x u/1, WT x u/1
  Effective Total weight of car/1(effective total weight of car) -> (0.5xWeffective x lm/L)-(deltaWy x 0.375)1/2(effective total weight of car), (0.5xWeffective x lm/L)+(deltaWy x 0.375)/2(effective total weight of car), effective weight of one front wheel/1(In1), WT x u/2  "effective total weight of car"
  Lateral weight transfer (deltaWy) x 0.625/1 -> (0.5xWeffective x (L-lm)/L)-(deltaWy x 0.625)1/2, (0.5xWeffective x (L-lm)/L)+(deltaWy x 0.625)/1
  62.5% of this weight tranfer/1 -> Lateral weight transfer (deltaWy) x 0.625/2
  Lateral weight transfer (deltaWy)=(FxHm)/T/1(Lateral weight transfer (deltaWy)) -> Product/1, Lateral weight transfer (deltaWy) x 0.625/1
  L/1 -> (0.5xWeffective x lm/L)-(deltaWy x 0.375)1/3(L), (0.5xWeffective x lm/L)+(deltaWy x 0.375)/3(L), front wheel load bearing ratio (L-lm)/L/1(In1)
  Weight (W)/1 -> Effective Total weight of car/2(In2)
  Wrovert x u/1 -> Rear outer wheel design cornering force (Wrolat)/1  "Rear outer design cornering force (Wrolat)"
  Hm/1 -> Lateral weight transfer (deltaWy)=(FxHm)/T/1(Hm)
  effective weight of one front wheel/1(effective weight of one front wheel) -> (0.5xWeffective x (L-lm)/L)-(deltaWy x 0.625)1/1, (0.5xWeffective x (L-lm)/L)+(deltaWy x 0.625)/2
  Rear outer vertical wheel load x maximum cornering DMF/1 -> Wrovert x u/1  "Weight vertical of rear outer wheel(Wrovert)"
  In1/1 -> Front inner vertical wheel load x maximum cornering DMF/1, Front outer vertical wheel load x maximum cornering DMF/1, Rear outer vertical wheel load x maximum cornering DMF/2, Rear inner vertical wheel load x maximum cornering DMF/1
  Max Downforce Multiplication Factor/1 -> Effective Total weight of car/1(In1)
  (0.5xWeffective x (L-lm)/L)+(deltaWy x 0.625)/1 -> Front outer vertical wheel load x maximum cornering DMF/2  "Front outer vertical wheel load"
  WT x u/1 -> Lateral weight transfer (deltaWy)=(FxHm)/T/2(In2)  "Maximum breaking force(F)"
  (0.5xWeffective x lm/L)+(deltaWy x 0.375)/1(Rear outer vertical wheel load) -> Rear outer vertical wheel load x maximum cornering DMF/1  "rear outer vertical wheel load"
  front wheel load bearing ratio (L-lm)/L/1(Out1) -> effective weight of one front wheel/2(front wheel load bearing ratio (L-lm)/L)  "front wheel load bearing ratio (L-lm)/L"
  Front outer vertical wheel load x maximum cornering DMF/1 -> Wfovert x u/2  "Weight vertical of front outer wheel(Wfovert)"
  Wfovert x u/1 -> Front outer wheel design cornering force (Wfolat)/1  "Front outer design cornering force (Wfolat)"
  T/1 -> Lateral weight transfer (deltaWy)=(FxHm)/T/3(T)
  "37.5% of this weight tranfer "/1 -> Product/2
  Product/1 -> (0.5xWeffective x lm/L)-(deltaWy x 0.375)1/1(In1), (0.5xWeffective x lm/L)+(deltaWy x 0.375)/1(In1)
  (0.5xWeffective x lm/L)-(deltaWy x 0.375)1/1(Rear inner vertical wheel load) -> Rear inner vertical wheel load x maximum cornering DMF/2  "rear inner vertical wheel load"
  Wrivert x u/1 -> Rear outer wheel design cornering force (Wrilat) [smaller force expericned]/1  "Rear inner design cornering force (Wrilat)"
  Rear inner vertical wheel load x maximum cornering DMF/1 -> Wrivert x u/1  "Weight vertical of reart outer wheel(Wrivert)"
  (0.5xWeffective x (L-lm)/L)-(deltaWy x 0.625)1/1 -> Front inner vertical wheel load x maximum cornering DMF/2  "Front inner vertical wheel load"
  Front inner vertical wheel load x maximum cornering DMF/1 -> Wfivert x u/2  "Weight vertical of front inner wheel(Wfivert)"
  Wfivert x u/1 -> Front inner wheel design cornering force (Wfilat) [smaller forces experienced]/1  "Front inner design cornering force (Wfilat)"

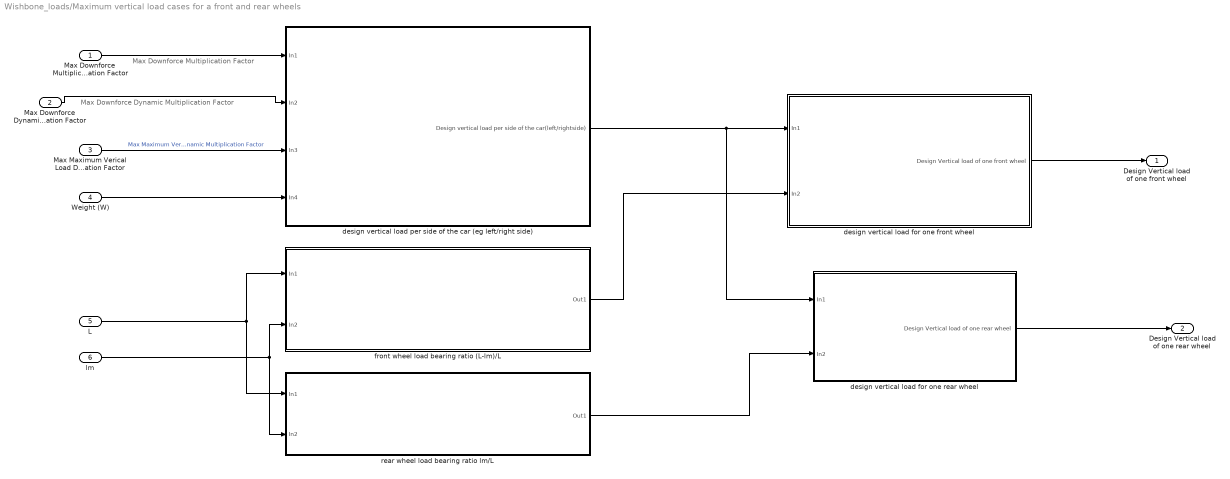
== system Wishbone_loads/Maximum vertical load cases for a front and rear wheels ==
  note: Max Downforce Dynamic Multiplication Factor
  note: Max Downforce Multiplication Factor
  Max Downforce Multiplication Factor : Inport
  Max Downforce Dynamic Multiplication Factor : Inport  Port=2
  Max Maximum Verical Load Dynamic Multiplication Factor : Inport  Port=3
  Weight (W) : Inport  Port=4
  L : Inport  Port=5
  lm : Inport  Port=6
  design vertical load for one front wheel : Subsystem
  design vertical load for one rear wheel : Subsystem
  design vertical load per side of the car (eg left/right side) : Subsystem
  front wheel load bearing ratio (L-lm)/L : Subsystem
  rear wheel load bearing ratio lm/L : Subsystem
  Design Vertical load of one front wheel : Outport
  Design Vertical load of one rear wheel : Outport  Port=2
  wires:
  Max Downforce Multiplication Factor/1 -> design vertical load per side of the car (eg left/right side)/1(In1)
  front wheel load bearing ratio (L-lm)/L/1(Out1) -> design vertical load for one front wheel/2(In2)
  lm/1 -> rear wheel load bearing ratio lm/L/2(In2), front wheel load bearing ratio (L-lm)/L/2(In2)
  L/1 -> rear wheel load bearing ratio lm/L/1(In1), front wheel load bearing ratio (L-lm)/L/1(In1)
  Weight (W)/1 -> design vertical load per side of the car (eg left/right side)/4(In4)
  design vertical load per side of the car (eg left/right side)/1(Design vertical load per side of the car(left/rightside)) -> design vertical load for one front wheel/1(In1), design vertical load for one rear wheel/1(In1)
  rear wheel load bearing ratio lm/L/1(Out1) -> design vertical load for one rear wheel/2(In2)
  Max Downforce Dynamic Multiplication Factor/1 -> design vertical load per side of the car (eg left/right side)/2(In2)
  Max Maximum Verical Load Dynamic Multiplication Factor/1 -> design vertical load per side of the car (eg left/right side)/3(In3)  "Max Maximum Verical Load Dynamic Multiplication Factor"
  design vertical load for one rear wheel/1(Design Vertical load of one rear wheel) -> Design Vertical load of one rear wheel/1
  design vertical load for one front wheel/1(Design Vertical load of one front wheel) -> Design Vertical load of one front wheel/1

== system Wishbone_loads/For Centre of Mass not at centre of car Lateral load Transfer-each wheel/(Aalpha x cos(alpha))- sin(alpha)) ==
  In1 : Inport
  In2 : Inport  Port=2
  (Aalpha x cos(alpha))- sin(alpha)) : Sum  Inputs=+-
  Aalpha x cos(alpha) : Product
  Cosine : simulink/Lookup Tables/Cosine  Formula=cos(2*pi*u)  NumDataPoints=(2^5)+1  OutputWordLength=16  InternalRulePriority=Speed
  Sine : simulink/Lookup Tables/Sine  Formula=sin(2*pi*u)  NumDataPoints=(2^5)+1  OutputWordLength=16  InternalRulePriority=Speed
  "Ay=lateral acceleration, measured in gs" : Outport
  wires:
  Aalpha x cos(alpha)/1 -> (Aalpha x cos(alpha))- sin(alpha))/1
  In2/1 -> Cosine/1, Sine/1
  Sine/1 -> (Aalpha x cos(alpha))- sin(alpha))/2
  Cosine/1 -> Aalpha x cos(alpha)/2
  In1/1 -> Aalpha x cos(alpha)/1
  (Aalpha x cos(alpha))- sin(alpha))/1 -> "Ay=lateral acceleration, measured in gs"/1  "Ay=lateral acceleration, measured in gs"

== system Wishbone_loads/For Centre of Mass not at centre of car Lateral load Transfer-each wheel/V^2//(Rg) ==
  In1 : Inport
  In2 : Inport  Port=2
  In3 : Inport  Port=3
  Rg : Product
  V^2 : Product
  V^2/(Rg) : Product  Inputs=*/
  Aalpha=centrifugal acceleration (measusred in g's) : Outport
  wires:
  In1/1 -> V^2/2, V^2/1
  Rg/1 -> V^2/(Rg)/2
  In3/1 -> Rg/2
  V^2/(Rg)/1 -> Aalpha=centrifugal acceleration (measusred in g's)/1  "Aalpha=centrifugal acceleration"
  In2/1 -> Rg/1
  V^2/1 -> V^2/(Rg)/1

== system Wishbone_loads/For Centre of Mass not at centre of car Lateral load Transfer-each wheel/W(Aalpha x sin(alpha)) +cos(alpha)) ==
  Weight (W) : Inport
  Aalpha=centrifugal acceleration (measusred in g's) : Inport  Port=2
  u : Inport  Port=3
  (Aalpha x sin(alpha)) +cos(alpha)) : Sum
  Aalpha x sin(alpha) : Product
  Cosine : simulink/Lookup Tables/Cosine  Formula=cos(2*pi*u)  NumDataPoints=(2^5)+1  OutputWordLength=16  InternalRulePriority=Speed
  Sine : simulink/Lookup Tables/Sine  Formula=sin(2*pi*u)  NumDataPoints=(2^5)+1  OutputWordLength=16  InternalRulePriority=Speed
  W(Aalpha x sin(alpha)) +cos(alpha)) : Product
  W’ = effective weight due to bank angle and speed : Outport
  wires:
  Aalpha=centrifugal acceleration (measusred in g's)/1 -> Aalpha x sin(alpha)/1
  W(Aalpha x sin(alpha)) +cos(alpha))/1 -> W’ = effective weight due to bank angle and speed/1  "W’ = effective weight due to bank angle and speed"
  Weight (W)/1 -> W(Aalpha x sin(alpha)) +cos(alpha))/2
  Aalpha x sin(alpha)/1 -> (Aalpha x sin(alpha)) +cos(alpha))/1
  Cosine/1 -> (Aalpha x sin(alpha)) +cos(alpha))/2
  u/1 -> Cosine/1, Sine/1
  (Aalpha x sin(alpha)) +cos(alpha))/1 -> W(Aalpha x sin(alpha)) +cos(alpha))/1  "Ay=lateral acceleration, measured in gs"
  Sine/1 -> Aalpha x sin(alpha)/2

== system Wishbone_loads/Maximum Vertical Loads-For Centre of Mass not at centre of car Longitudinal load transfer-each wheel /(W)(h//l)Ax ==
  In1 : Inport
  In2 : Inport  Port=2
  In3 : Inport  Port=3
  In4 : Inport  Port=4
  (W)(h/l)Ax : Product
  Ax(h/l) : Product
  h/l : Product  Inputs=*/
  Out1 : Outport
  wires:
  In4/1 -> Ax(h/l)/2
  h/l/1 -> Ax(h/l)/1
  In1/1 -> (W)(h/l)Ax/1
  In2/1 -> h/l/1
  (W)(h/l)Ax/1 -> Out1/1
  In3/1 -> h/l/2
  Ax(h/l)/1 -> (W)(h/l)Ax/2

== system Wishbone_loads/Maximum Vertical Loads-For Centre of Mass not at centre of car Longitudinal load transfer-each wheel /+Cx3(W)(h//l)Ax ==
  Cx3 : Inport
  (W)(h/l)Ax : Inport  Port=2
  Cx3(W)(h/l)Ax : Product
  DeltaW3 : Outport
  wires:
  Cx3(W)(h/l)Ax/1 -> DeltaW3/1  "DeltaW3"
  Cx3/1 -> Cx3(W)(h/l)Ax/2
  (W)(h/l)Ax/1 -> Cx3(W)(h/l)Ax/1

== system Wishbone_loads/Maximum Vertical Loads-For Centre of Mass not at centre of car Longitudinal load transfer-each wheel /+Cx4(W)(h//l)Ax  ==
  Cx4 : Inport
  (W)(h/l)Ax : Inport  Port=2
  Cx4(W)(h/l)Ax : Product
  DeltaW4 : Outport
  wires:
  Cx4(W)(h/l)Ax/1 -> DeltaW4/1  "DeltaW4"
  Cx4/1 -> Cx4(W)(h/l)Ax/2
  (W)(h/l)Ax/1 -> Cx4(W)(h/l)Ax/1

== system Wishbone_loads/Maximum Vertical Loads-For Centre of Mass not at centre of car Longitudinal load transfer-each wheel /-Cx1(W)(h//l)Ax ==
  Cx1 : Inport
  (W)(h/l)Ax : Inport  Port=2
  -Cx1 : Product
  Constant : Constant  Value=-1
  Cx1(W)(h/l)Ax : Product
  DeltaW1 : Outport
  wires:
  Cx1(W)(h/l)Ax/1 -> DeltaW1/1  "DeltaW1"
  Cx1/1 -> -Cx1/2
  (W)(h/l)Ax/1 -> Cx1(W)(h/l)Ax/1
  Constant/1 -> -Cx1/1
  -Cx1/1 -> Cx1(W)(h/l)Ax/2

== system Wishbone_loads/Maximum Vertical Loads-For Centre of Mass not at centre of car Longitudinal load transfer-each wheel /-Cx2(W)(h//l)Ax  ==
  Cx2 : Inport
  (W)(h/l)Ax : Inport  Port=2
  -Cx2 : Product
  Constant : Constant  Value=-1
  Cx2(W)(h/l)Ax : Product
  DeltaW2 : Outport
  wires:
  Cx2(W)(h/l)Ax/1 -> DeltaW2/1  "DeltaW2"
  Cx2/1 -> -Cx2/2
  (W)(h/l)Ax/1 -> Cx2(W)(h/l)Ax/1
  Constant/1 -> -Cx2/1
  -Cx2/1 -> Cx2(W)(h/l)Ax/2

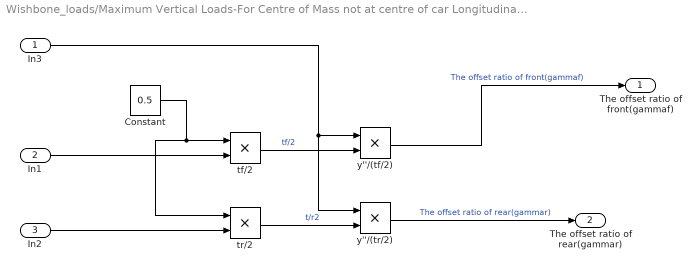
== system Wishbone_loads/Maximum Vertical Loads-For Centre of Mass not at centre of car Longitudinal load transfer-each wheel /Subsystem ==
  In3 : Inport
  In1 : Inport  Port=2
  In2 : Inport  Port=3
  Constant : Constant  Value=0.5
  tf/2 : Product
  tr/2 : Product
  y''/(tf/2) : Product
  y''/(tr/2) : Product
  The offset ratio of front(gammaf) : Outport
  The offset ratio of rear(gammar) : Outport  Port=2
  wires:
  tf/2/1 -> y''/(tf/2)/2  "tf/2"
  In1/1 -> tf/2/2
  In3/1 -> y''/(tr/2)/1, y''/(tf/2)/1
  tr/2/1 -> y''/(tr/2)/2  "t/r2"
  Constant/1 -> tr/2/1, tf/2/1
  y''/(tf/2)/1 -> The offset ratio of front(gammaf)/1  "The offset ratio of front(gammaf)"
  In2/1 -> tr/2/2
  y''/(tr/2)/1 -> The offset ratio of rear(gammar)/1  "The offset ratio of rear(gammar)"

== system Wishbone_loads/Maximum Vertical Loads-For Centre of Mass not at centre of car Longitudinal load transfer-each wheel /Subsystem1 ==
  In1 : Inport
  (1+gammaf) : Sum
  (1-gammaf) : Sum  Inputs=+-
  Constant1 : Constant
  (1+gammaf)1 : Outport
  (1-gammaf)1 : Outport  Port=2
  wires:
  (1-gammaf)/1 -> (1-gammaf)1/1  "(1-gammaf)"
  Constant1/1 -> (1-gammaf)/1, (1+gammaf)/2
  In1/1 -> (1+gammaf)/1, (1-gammaf)/2
  (1+gammaf)/1 -> (1+gammaf)1/1  "(1+gammaf)"

== system Wishbone_loads/Maximum Vertical Loads-For Centre of Mass not at centre of car Longitudinal load transfer-each wheel /Subsystem2 ==
  The offset ratio of rear(gammar) : Inport
  (1+gammaf) : Sum
  (1-gammaf) : Sum  Inputs=+-
  Constant1 : Constant
  (1+gammaf)1 : Outport
  (1-gammaf)1 : Outport  Port=2
  wires:
  (1-gammaf)/1 -> (1-gammaf)1/1  "(1-gammaf)"
  Constant1/1 -> (1-gammaf)/1, (1+gammaf)/2
  The offset ratio of rear(gammar)/1 -> (1+gammaf)/1, (1-gammaf)/2
  (1+gammaf)/1 -> (1+gammaf)1/1  "(1+gammaf)"

== system Wishbone_loads/Maximum Vertical Loads-For Centre of Mass not at centre of car Longitudinal load transfer-each wheel /Subsystem3 ==
  In1 : Inport
  In2 : Inport  Port=2
  Constant : Constant  Value=0.5
  "½ (1+gammaf) " : Product
  ½ (1+gammaf) 1 : Product
  Cx1 : Outport
  Cx2 : Outport  Port=2
  wires:
  Constant/1 -> "½ (1+gammaf) "/2, ½ (1+gammaf) 1/1
  ½ (1+gammaf) 1/1 -> Cx2/1  "Cx2"
  "½ (1+gammaf) "/1 -> Cx1/1  "Cx1"
  In2/1 -> ½ (1+gammaf) 1/2
  In1/1 -> "½ (1+gammaf) "/1

== system Wishbone_loads/Maximum Vertical Loads-For Centre of Mass not at centre of car Longitudinal load transfer-each wheel /Subsystem4 ==
  In1 : Inport
  In2 : Inport  Port=2
  Constant : Constant  Value=0.5
  "½ (1+gammaf) " : Product
  ½ (1+gammaf) 1 : Product
  Cx3 : Outport
  Cx4 : Outport  Port=2
  wires:
  Constant/1 -> "½ (1+gammaf) "/2, ½ (1+gammaf) 1/1
  ½ (1+gammaf) 1/1 -> Cx4/1  "Cx4"
  "½ (1+gammaf) "/1 -> Cx3/1  "Cx3"
  In2/1 -> ½ (1+gammaf) 1/2
  In1/1 -> "½ (1+gammaf) "/1

== system Wishbone_loads/Maximum Vertical Loads-For Centre of Mass not at centre of car Longitudinal load transfer-each wheel /V^2//(Rg) ==
  In1 : Inport
  In2 : Inport  Port=2
  In3 : Inport  Port=3
  Rg : Product
  V^2 : Product
  V^2/(Rg) : Product  Inputs=*/
  Aalpha=centrifugal acceleration (measusred in g's) : Outport
  wires:
  In1/1 -> V^2/2, V^2/1
  Rg/1 -> V^2/(Rg)/2
  In3/1 -> Rg/2
  V^2/(Rg)/1 -> Aalpha=centrifugal acceleration (measusred in g's)/1  "Aalpha=centrifugal acceleration"
  In2/1 -> Rg/1
  V^2/1 -> V^2/(Rg)/1

== system Wishbone_loads/Maximum Vertical Loads-For Centre of Mass not at centre of car Longitudinal load transfer-each wheel /W(Aalpha x sin(alpha)) +cos(alpha)) ==
  Weight (W) : Inport
  Aalpha=centrifugal acceleration (measusred in g's) : Inport  Port=2
  u : Inport  Port=3
  (Aalpha x sin(alpha)) +cos(alpha)) : Sum
  Aalpha x sin(alpha) : Product
  Cosine : simulink/Lookup Tables/Cosine  Formula=cos(2*pi*u)  NumDataPoints=(2^5)+1  OutputWordLength=16  InternalRulePriority=Speed
  Sine : simulink/Lookup Tables/Sine  Formula=sin(2*pi*u)  NumDataPoints=(2^5)+1  OutputWordLength=16  InternalRulePriority=Speed
  W(Aalpha x sin(alpha)) +cos(alpha)) : Product
  W’ = effective weight due to bank angle and speed : Outport
  wires:
  Aalpha=centrifugal acceleration (measusred in g's)/1 -> Aalpha x sin(alpha)/1
  W(Aalpha x sin(alpha)) +cos(alpha))/1 -> W’ = effective weight due to bank angle and speed/1  "W’ = effective weight due to bank angle and speed"
  Weight (W)/1 -> W(Aalpha x sin(alpha)) +cos(alpha))/2
  Aalpha x sin(alpha)/1 -> (Aalpha x sin(alpha)) +cos(alpha))/1
  Cosine/1 -> (Aalpha x sin(alpha)) +cos(alpha))/2
  u/1 -> Cosine/1, Sine/1
  (Aalpha x sin(alpha)) +cos(alpha))/1 -> W(Aalpha x sin(alpha)) +cos(alpha))/1  "Ay=lateral acceleration, measured in gs"
  Sine/1 -> Aalpha x sin(alpha)/2

== system Wishbone_loads/Maximum acceleraton load cases for a front and rear wheel/Front wheel loads(Wfl and Wfr)=(Wr- deltaWx)//2 ==
  L : Inport
  Static front axle load(Wf) : Inport  Port=2
  rear wheels Traction Force(Fr) : Inport  Port=3
  Hm : Inport  Port=4
  (Wr - deltaWx)/2 : Product
  Constant : Constant  Value=0.5
  Longitudinal weight transfer (deltaWx)=(FrxHm)/L : Subsystem
  Wr - deltaWx : Sum  Inputs=+-
  Front wheel loads(Wfl/Wfr) : Outport
  wires:
  Constant/1 -> (Wr - deltaWx)/2/2
  L/1 -> Longitudinal weight transfer (deltaWx)=(FrxHm)/L/3(L)
  Static front axle load(Wf)/1 -> Wr - deltaWx/1
  Wr - deltaWx/1 -> (Wr - deltaWx)/2/1
  Longitudinal weight transfer (deltaWx)=(FrxHm)/L/1(Longitudinal weight transfer (deltaWx)) -> Wr - deltaWx/2
  rear wheels Traction Force(Fr)/1 -> Longitudinal weight transfer (deltaWx)=(FrxHm)/L/2(Traction Force(Fr))
  Hm/1 -> Longitudinal weight transfer (deltaWx)=(FrxHm)/L/1(Hm)
  (Wr - deltaWx)/2/1 -> Front wheel loads(Wfl/Wfr)/1  "front wheel loads(Wfl/ Wfr)"

== system Wishbone_loads/Maximum acceleraton load cases for a front and rear wheel/Rear wheel loads(Wrl and Wrr)=(Wr+ deltaWx)//2 ==
  L : Inport
  In2 : Inport  Port=2
  rear wheels Traction Force(F) : Inport  Port=3
  Hm : Inport  Port=4
  (Wr + deltaWx)/2 : Product
  Constant : Constant  Value=0.5
  Longitudinal weight transfer (deltaWx)=(FxHm)/L : Subsystem
  Wr + deltaWx : Sum
  Rear wheel load(Wrl/Wrr) : Outport
  wires:
  Constant/1 -> (Wr + deltaWx)/2/2
  L/1 -> Longitudinal weight transfer (deltaWx)=(FxHm)/L/3(L)
  In2/1 -> Wr + deltaWx/1
  Wr + deltaWx/1 -> (Wr + deltaWx)/2/1
  Longitudinal weight transfer (deltaWx)=(FxHm)/L/1(Longitudinal weight transfer (deltaWx)) -> Wr + deltaWx/2
  rear wheels Traction Force(F)/1 -> Longitudinal weight transfer (deltaWx)=(FxHm)/L/2(Traction Force(F))
  Hm/1 -> Longitudinal weight transfer (deltaWx)=(FxHm)/L/1(Hm)
  (Wr + deltaWx)/2/1 -> Rear wheel load(Wrl/Wrr)/1  "Rear wheel loads(Wrl/ Wrr)"
